simulink model "nonlinear_model"  (R2020b)
settings: Solver=ode23t  StartTime=0.0  StopTime=20  MaxStep=0.05  RelTol=1e-3
values from neighbouring files (symbols this model uses):
  par = readtable("parameters.xlsx", opts, "UseExcel", false)    [identification.m]
settings Model: Creator=emiel  LastModifiedBy=emiel

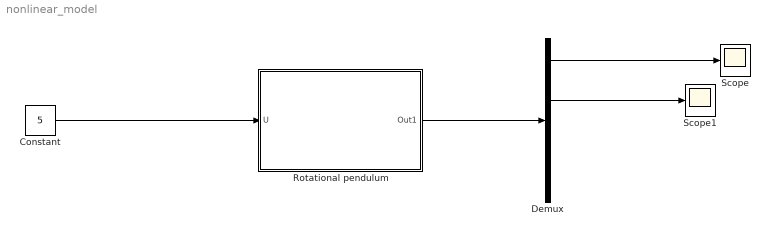
== system nonlinear_model ==
  Constant : Constant  Value=5
  Demux : Demux
  Rotational pendulum : Subsystem
  Scope : Scope
  Scope1 : Scope
  wires:
  Constant/1 -> Rotational pendulum/1(U)
  Rotational pendulum/1(Out1) -> Demux/1
  Demux/1 -> Scope/1
  Demux/2 -> Scope1/1

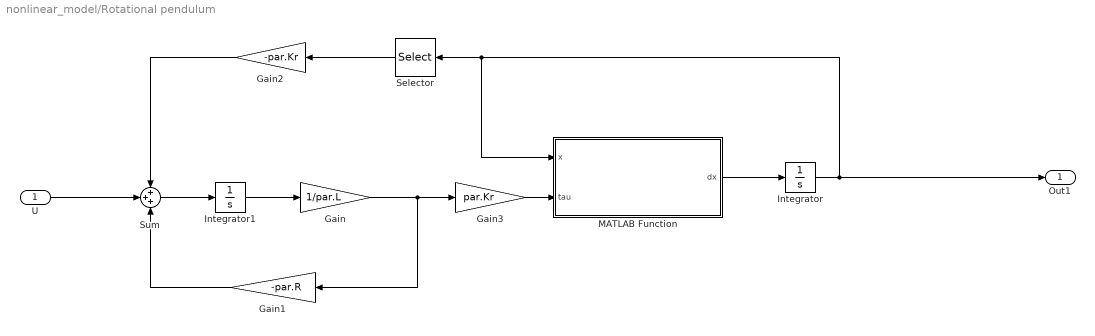
== system nonlinear_model/Rotational pendulum ==
  U : Inport
  Gain : Gain  Gain=1/par.L
  Gain1 : Gain  Gain=-par.R
  Gain2 : Gain  Gain=-par.Kr
  Gain3 : Gain  Gain=par.Kr
  Integrator : Integrator
  Integrator1 : Integrator
  MATLAB Function : MATLAB Function  TreatAsAtomicUnit=on
  Selector : Selector  InputPortWidth=4  IndexOptions=Index vector (dialog)  Indices=[3]  OutputSizes=1
  Sum : Sum  Inputs=+++
  Out1 : Outport
  wires:
  MATLAB Function/1(dx) -> Integrator/1
  Integrator/1 -> MATLAB Function/1(x), Selector/1, Out1/1
  Gain/1 -> Gain3/1, Gain1/1
  Integrator1/1 -> Gain/1
  Sum/1 -> Integrator1/1
  Gain1/1 -> Sum/3
  Selector/1 -> Gain2/1
  Gain2/1 -> Sum/1
  Gain3/1 -> MATLAB Function/2(tau)
  U/1 -> Sum/2

== matlab function nonlinear_model/Rotational pendulum/MATLAB Function ==
  data: x input size=4; tau input size=1; dx output size=4; par parameter
function dx = pendulum_dynamics(x, tau, par)

    % x = [theta1, theta2, dtheta1, dtheta2
    
    d1 = par.d1;
    d2 = par.d2;
    l1 = par.l1;
    l2 = par.l2;
    I1 = par.I1;
    I2 = par.I2;
    Iball = par.Iball;
    m1 = par.m1;
    m2 = par.m2;
    mball = par.mball;
    g = par.g;
    
    theta1 = x(1);
    theta2 = x(2);
    theta1_dot = x(3);
    theta2_dot = x(4);
    
    mass = [1, 0, 0, 0; ...
            0, 1, 0, 0; ...
            0, 0, I1 + I2 + Iball + d1^2*m1 + m2*(2*d2^2 + 4*d2*l1*cos(theta2) + 2*l1^2)/2 + mball*(2*l1^2 + 4*l1*l2*cos(theta2) + 2*l2^2)/2, I2 + Iball + m2*(2*d2^2 + 2*d2*l1*cos(theta2))/2 + mball*(2*l1*l2*cos(theta2) + 2*l2^2)/2; ...
            0, 0, I2 + Iball + m2*(2*d2^2 + 2*d2*l1*cos(theta2))/2 + mball*(2*l1*l2*cos(theta2) + 2*l2^2)/2, I2 + Iball + d2^2*m2 + l2^2*mball];

    forcing = [theta1_dot; ...
               theta2_dot; ...
               -d1*g*m1*sin(theta1) - g*m2*(-d2*(-sin(theta1)*cos(theta2) - sin(theta2)*cos(theta1)) + l1*sin(theta1)) - g*mball*(l1*sin(theta1) - l2*(-sin(theta1)*cos(theta2) - sin(theta2)*cos(theta1))) - m2*(-2*d2*l1*(theta1_dot + theta2_dot)*sin(theta2)*theta2_dot - 2*d2*l1*sin(theta2)*theta1_dot*theta2_dot)/2 - mball*(-2*l1*l2*(theta1_dot + theta2_dot)*sin(theta2)*theta2_dot - 2*l1*l2*sin(theta2)*theta1_dot*theta2_dot)/2 + tau; ...
               d2*g*m2*(-sin(theta1)*cos(theta2) - sin(theta2)*cos(theta1)) - d2*l1*m2*(theta1_dot + theta2_dot)*sin(theta2)*theta1_dot + d2*l1*m2*sin(theta2)*theta1_dot*theta2_dot + g*l2*mball*(-sin(theta1)*cos(theta2) - sin(theta2)*cos(theta1)) - l1*l2*mball*(theta1_dot + theta2_dot)*sin(theta2)*theta1_dot + l1*l2*mball*sin(theta2)*theta1_dot*theta2_dot];

           
    dx = mass\forcing;
